simulink model "SHE_bipolar_HB"  (R2023a)
settings: Solver=ode45  StartTime=0.0  StopTime=2  MaxStep=1e-4  RelTol=1e-3
undefined symbols (not defined in the file): t0, t1, t2
libraries: spsDCVoltageSourceLib x2, spsMosfetLib x2, simulink x1, spsSeriesRLCBranchLib x1, spsVoltageMeasurementLib x1, sps_lib x1
settings Model: Creator=Blu-Ray  LastModifiedBy=Blu-Ray

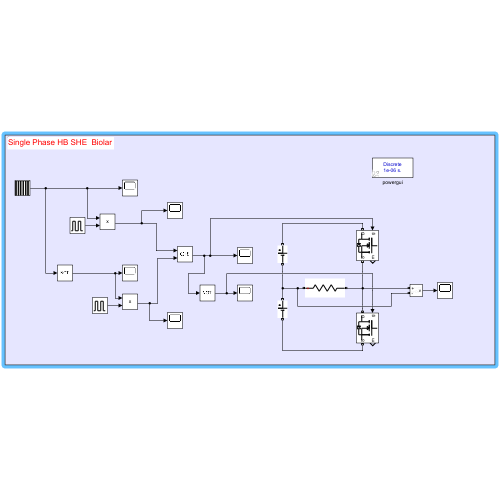
[thumbnail: Simulink's stored preview of the top-level diagram]
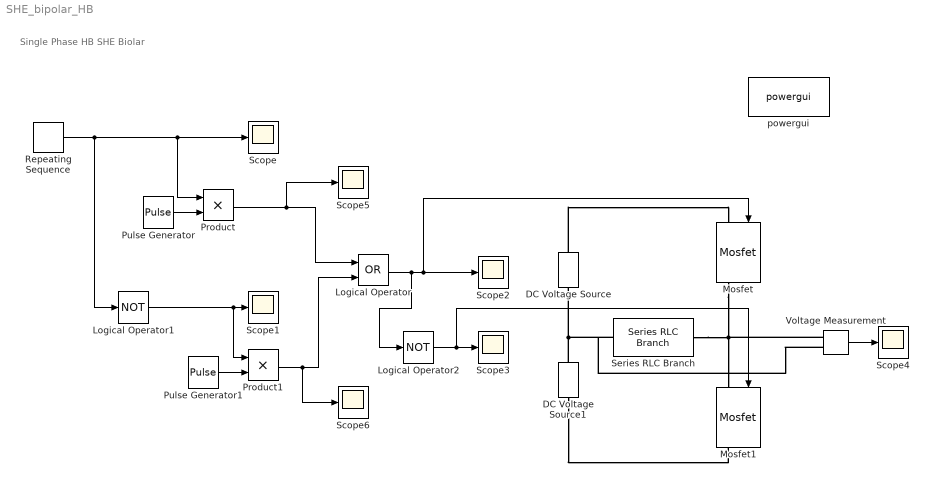
== system SHE_bipolar_HB ==
  note: Single Phase HB SHE Biolar
  DC Voltage Source : spsDCVoltageSourceLib/DC Voltage Source  Amplitude=100  Measurements=None
  DC Voltage Source1 : spsDCVoltageSourceLib/DC Voltage Source  Amplitude=100  Measurements=None
  Logical Operator : Logic  Operator=OR  AllPortsSameDT=off  OutDataTypeStr=boolean
  Logical Operator1 : Logic  Operator=NOT  AllPortsSameDT=off  OutDataTypeStr=boolean
  Logical Operator2 : Logic  Operator=NOT  AllPortsSameDT=off  OutDataTypeStr=boolean
  Mosfet : spsMosfetLib/Mosfet  Ron=0.1  Lon=0  Rd=0.01  Vfd=0  IC=0  Rs=1e5  Cs=inf  Measurements=on
  Mosfet1 : spsMosfetLib/Mosfet  Ron=0.1  Lon=0  Rd=0.01  Vfd=0  IC=0  Rs=1e5  Cs=inf  Measurements=on
  Product : Product
  Product1 : Product
  Pulse Generator : DiscretePulseGenerator  PulseType=Time based  Period=.02  PulseWidth=50
  Pulse Generator1 : DiscretePulseGenerator  PulseType=Time based  Period=.02  PulseWidth=50  PhaseDelay=0.01
  Repeating Sequence : simulink/Sources/Repeating Sequence  rep_seq_t="[0 t1 t1+t0 t2 t2+t0 0.01/2+t1  0.01/2+t1+t0 0.01/2+t2 0.01/2+t2+t0 0.01]"  rep_seq_y=[1 1 0 0 1 1 0 0 1 1]
  Scope{,1..6} (7 alike) : Scope
  Series RLC Branch : spsSeriesRLCBranchLib/Series RLC Branch  LConnTagsString=__new0  RConnTagsString=__new0  BranchType=R  Resistance=10  Inductance=1e-3  SetiL0=off  InitialCurrent=0  Capacitance=1e-6  Setx0=off  InitialVoltage=0  Measurements=None
  Voltage Measurement : spsVoltageMeasurementLib/Voltage Measurement  PhasorSimulation=off  OutputType=Complex  PSBequivalent=0
  powergui : sps_lib/powergui  Priority=1  SimulationMode=Discrete  SampleTime=1e-6  frequency=60  Iterations=50  frequencyindice=0  Pbase=100e6  ErrMax=1e-4  UnitsV=kV  UnitsW=MW  buscounter=0  FunctionMessages=off  echomessages=off  EnableUseOfTLC=off  CurrentSourceSwitches=off  DisableSnubberDevices=off  DisableRonSwitches=off  DisableVfSwitches=off  DisplayEquations=off  AutomaticDiscreteSolvers=off  SolverType=Tustin/Backward Euler (TBE)  Interpol=off  ExternalGateDelay=off  methode=off  Ts=100  x0status=blocks  SPID=on  SwTol=0  HookPort=off  NonlinearTolerance=1e-4  nMaxIteration=100  ContinueOnMaxIteration=off  RestoreLinks=warning  ResistiveCurrentMeasurement=off  Frange=[0:2:500]  Ylog=off  Xlog=on  ShowGrid=off  save=off  variable=ZData  structure=0  ZoomFFT=off  StartTime=0.0  cycles=1  DisplayStyle=1  fundamental=60  FreqAxis=off  MaxFrequency=1000  frequencyindicesteady=1  RmsSteady=1  display=off
  wires:
  Logical Operator1/1 -> Product1/1, Scope1/1
  Repeating Sequence/1 -> Product/1, Scope/1, Logical Operator1/1
  Pulse Generator/1 -> Product/2
  Pulse Generator1/1 -> Product1/2
  Product/1 -> Scope5/1, Logical Operator/1
  Product1/1 -> Scope6/1, Logical Operator/2
  Logical Operator/1 -> Logical Operator2/1, Mosfet/1, Scope2/1
  Logical Operator2/1 -> Mosfet1/1, Scope3/1
  Voltage Measurement/1 -> Scope4/1
  connections:
  Mosfet/RConn1 -- Series RLC Branch/RConn1 -- Voltage Measurement/LConn1 -- Mosfet1/LConn1
  DC Voltage Source1/RConn1 -- Voltage Measurement/LConn2 -- Series RLC Branch/LConn1 -- DC Voltage Source/LConn1
  DC Voltage Source/RConn1 -- Mosfet/LConn1
  DC Voltage Source1/LConn1 -- Mosfet1/RConn1
